simulink subsystem "Read_PX4_Sensors"  (R2025a)
settings: Solver=VariableStepAuto  StartTime=0.0  StopTime=10.0  RelTol=1e-3
libraries: px4uORBlib x8
settings Model: Creator=gurt1  LastModifiedBy=gurt1
settings RTWCC: GPUComputeCapability=3.5

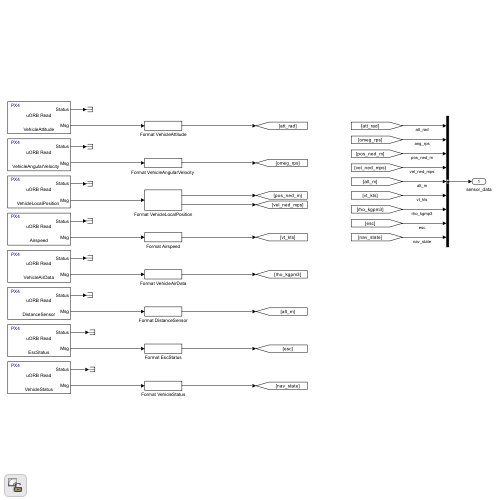
[thumbnail: Simulink's stored preview of the top-level diagram]
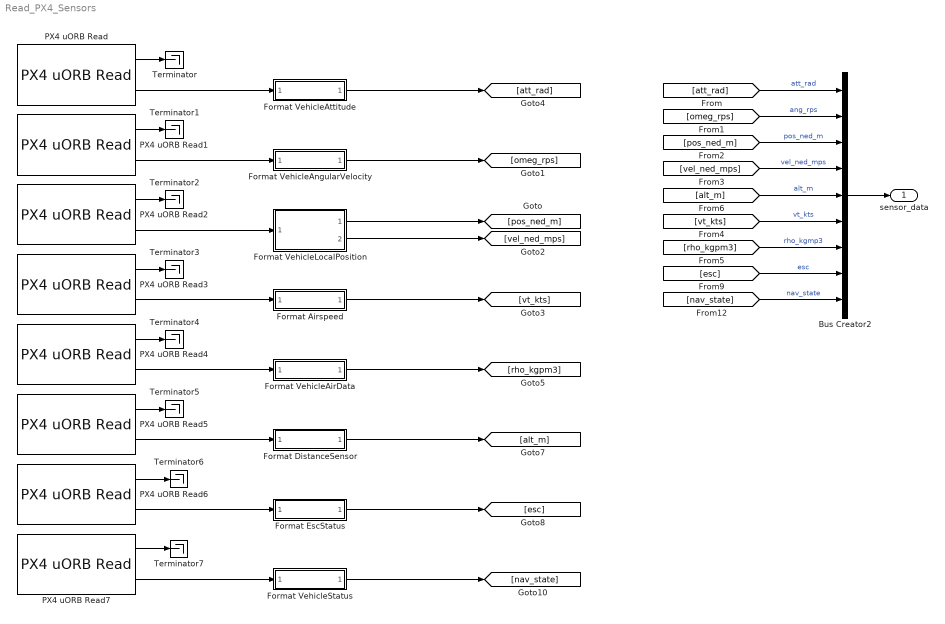
== system Read_PX4_Sensors ==
  Bus Creator2 : BusCreator  Inputs=9
  Format Airspeed : Subsystem
  Format DistanceSensor : Subsystem
  Format EscStatus : Subsystem
  Format VehicleAirData : Subsystem
  "Format VehicleAngularVelocity " : Subsystem
  Format VehicleAttitude : Subsystem
  Format VehicleLocalPosition : Subsystem
  Format VehicleStatus : Subsystem
  PX4 uORB Read : px4uORBlib/PX4 uORB Read  uORBTopic=VehicleAttitude  selectInstance=vehicle_attitude  SampleTime=-1  BlockingMode=off  BlockTimeout=1e-3
  PX4 uORB Read1 : px4uORBlib/PX4 uORB Read  uORBTopic=VehicleAngularVelocity  selectInstance=vehicle_angular_velocity  SampleTime=-1  BlockingMode=off  BlockTimeout=1e-3
  PX4 uORB Read2 : px4uORBlib/PX4 uORB Read  uORBTopic=VehicleLocalPosition  selectInstance=vehicle_local_position  SampleTime=-1  BlockingMode=off  BlockTimeout=1e-3
  PX4 uORB Read3 : px4uORBlib/PX4 uORB Read  uORBTopic=Airspeed  selectInstance=Airspeed  SampleTime=-1  BlockingMode=off  BlockTimeout=1e-3
  PX4 uORB Read4 : px4uORBlib/PX4 uORB Read  uORBTopic=VehicleAirData  selectInstance=VehicleAirData  SampleTime=-1  BlockingMode=off  BlockTimeout=1e-3
  PX4 uORB Read5 : px4uORBlib/PX4 uORB Read  uORBTopic=DistanceSensor  selectInstance=DistanceSensor  SampleTime=-1  BlockingMode=off  BlockTimeout=1e-3
  PX4 uORB Read6 : px4uORBlib/PX4 uORB Read  uORBTopic=EscStatus  selectInstance=EscStatus  SampleTime=-1  BlockingMode=off  BlockTimeout=1e-3
  PX4 uORB Read7 : px4uORBlib/PX4 uORB Read  uORBTopic=VehicleStatus  selectInstance=VehicleStatus  SampleTime=-1  BlockingMode=off  BlockTimeout=1e-3
  Terminator{,1..7} (8 alike) : Terminator
  sensor_data : Outport
  wires:
  PX4 uORB Read/1 -> Terminator/1
  Bus Creator2/1 -> sensor_data/1
  PX4 uORB Read1/1 -> Terminator1/1
  PX4 uORB Read2/1 -> Terminator2/1
  PX4 uORB Read3/1 -> Terminator3/1
  PX4 uORB Read4/1 -> Terminator4/1
  [att_rad] -> Bus Creator2/1  "att_rad"
  [omeg_rps] -> Bus Creator2/2  "ang_rps"
  [pos_ned_m] -> Bus Creator2/3  "pos_ned_m"
  [vel_ned_mps] -> Bus Creator2/4  "vel_ned_mps"
  [vt_kts] -> Bus Creator2/6  "vt_kts"
  [rho_kgpm3] -> Bus Creator2/7  "rho_kgmp3"
  PX4 uORB Read5/1 -> Terminator5/1
  [alt_m] -> Bus Creator2/5  "alt_m"
  PX4 uORB Read6/1 -> Terminator6/1
  [esc] -> Bus Creator2/8  "esc"
  PX4 uORB Read6/2 -> Format EscStatus/1(" ")
  Format EscStatus/1("   ") -> [esc]
  PX4 uORB Read7/1 -> Terminator7/1
  [nav_state] -> Bus Creator2/9  "nav_state"
  PX4 uORB Read/2 -> Format VehicleAttitude/1(" ")
  Format VehicleAttitude/1("  ") -> [att_rad]
  PX4 uORB Read1/2 -> "Format VehicleAngularVelocity "/1(" ")
  "Format VehicleAngularVelocity "/1("  ") -> [omeg_rps]
  PX4 uORB Read2/2 -> Format VehicleLocalPosition/1(" ")
  Format VehicleLocalPosition/1("  ") -> [pos_ned_m]
  Format VehicleLocalPosition/2("   ") -> [vel_ned_mps]
  PX4 uORB Read3/2 -> Format Airspeed/1(" ")
  Format Airspeed/1("  ") -> [vt_kts]
  PX4 uORB Read4/2 -> Format VehicleAirData/1(" ")
  Format VehicleAirData/1("  ") -> [rho_kgpm3]
  PX4 uORB Read5/2 -> Format DistanceSensor/1(" ")
  Format DistanceSensor/1("  ") -> [alt_m]
  PX4 uORB Read7/2 -> Format VehicleStatus/1(" ")
  Format VehicleStatus/1("  ") -> [nav_state]

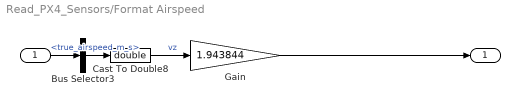
== system Read_PX4_Sensors/Format Airspeed ==
  " " : Inport
  Bus Selector3 : BusSelector  OutputSignals=true_airspeed_m_s
  Cast To Double8 : DataTypeConversion  OutDataTypeStr=double  SaturateOnIntegerOverflow=off  RndMeth=Floor
  Gain : Gain  Gain=1.943844
  "  " : Outport
  wires:
  Cast To Double8/1 -> Gain/1  "vz"
  " "/1 -> Bus Selector3/1
  Gain/1 -> "  "/1
  Bus Selector3/1 -> Cast To Double8/1  "<true_airspeed_m_s>"

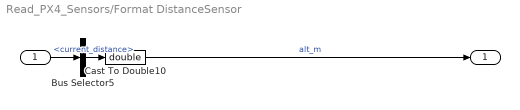
== system Read_PX4_Sensors/Format DistanceSensor ==
  " " : Inport
  Bus Selector5 : BusSelector  OutputSignals=current_distance
  Cast To Double10 : DataTypeConversion  OutDataTypeStr=double  SaturateOnIntegerOverflow=off  RndMeth=Floor
  "  " : Outport
  wires:
  Cast To Double10/1 -> "  "/1  "alt_m"
  Bus Selector5/1 -> Cast To Double10/1  "<current_distance>"
  " "/1 -> Bus Selector5/1

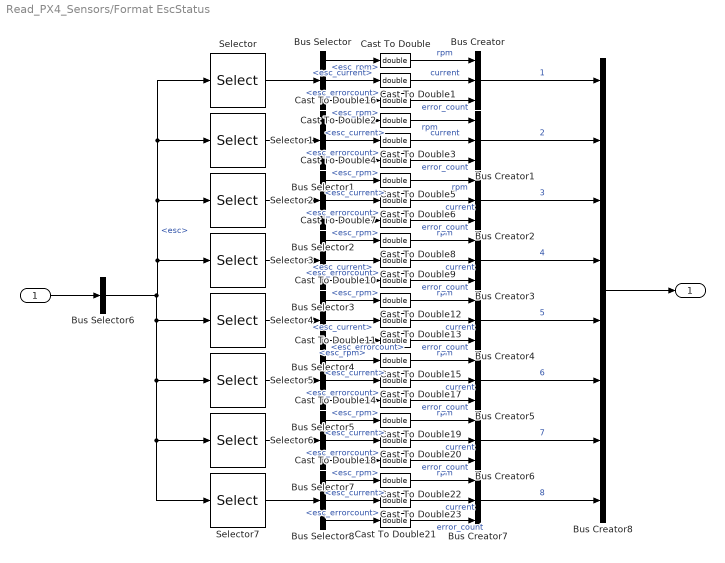
== system Read_PX4_Sensors/Format EscStatus ==
  " " : Inport
  Bus Creator{,1..7} (8 alike) : BusCreator  Inputs=3
  Bus Creator8 : BusCreator  Inputs=8
  Bus Selector{,1..5,7..8} (8 alike) : BusSelector  OutputSignals=esc_rpm,esc_current,esc_errorcount
  Bus Selector6 : BusSelector  OutputSignals=esc
  Cast To Double{,1..23} (24 alike) : DataTypeConversion  OutDataTypeStr=double  SaturateOnIntegerOverflow=off  RndMeth=Floor
  Selector : Selector  InputPortWidth=8  IndexOptions=Index vector (dialog)  Indices=[1]  OutputSizes=1
  Selector1 : Selector  InputPortWidth=8  IndexOptions=Index vector (dialog)  Indices=[2]  OutputSizes=1
  Selector2 : Selector  InputPortWidth=8  IndexOptions=Index vector (dialog)  Indices=[3]  OutputSizes=1
  Selector3 : Selector  InputPortWidth=8  IndexOptions=Index vector (dialog)  Indices=[4]  OutputSizes=1
  Selector4 : Selector  InputPortWidth=8  IndexOptions=Index vector (dialog)  Indices=[5]  OutputSizes=1
  Selector5 : Selector  InputPortWidth=8  IndexOptions=Index vector (dialog)  Indices=[6]  OutputSizes=1
  Selector6 : Selector  InputPortWidth=8  IndexOptions=Index vector (dialog)  Indices=[7]  OutputSizes=1
  Selector7 : Selector  InputPortWidth=8  IndexOptions=Index vector (dialog)  Indices=[8]  OutputSizes=1
  "   " : Outport
  wires:
  Selector3/1 -> Bus Selector3/1
  Bus Creator3/1 -> Bus Creator8/4  "4"
  Cast To Double22/1 -> Bus Creator7/1  "rpm"
  Bus Selector6/1 -> Selector/1, Selector1/1, Selector2/1, Selector3/1, Selector4/1, Selector5/1, Selector6/1, Selector7/1  "<esc>"
  Bus Selector1/1 -> Cast To Double2/1  "<esc_rpm>"
  Cast To Double13/1 -> Bus Creator4/2  "current"
  Bus Selector7/3 -> Cast To Double18/1  "<esc_errorcount>"
  Bus Creator7/1 -> Bus Creator8/8  "8"
  Cast To Double3/1 -> Bus Creator1/2  "current"
  Cast To Double18/1 -> Bus Creator6/3  "error_count"
  Bus Creator2/1 -> Bus Creator8/3  "3"
  Cast To Double15/1 -> Bus Creator5/1  "rpm"
  Cast To Double8/1 -> Bus Creator3/1  "rpm"
  Bus Selector5/3 -> Cast To Double14/1  "<esc_errorcount>"
  Cast To Double16/1 -> Bus Creator/3  "error_count"
  Cast To Double19/1 -> Bus Creator6/1  "rpm"
  Cast To Double9/1 -> Bus Creator3/2  "current"
  " "/1 -> Bus Selector6/1
  Selector2/1 -> Bus Selector2/1
  Cast To Double7/1 -> Bus Creator2/3  "error_count"
  Bus Selector8/1 -> Cast To Double22/1  "<esc_rpm>"
  Selector7/1 -> Bus Selector8/1
  Selector1/1 -> Bus Selector1/1
  Bus Selector2/3 -> Cast To Double7/1  "<esc_errorcount>"
  Bus Selector3/2 -> Cast To Double9/1  "<esc_current>"
  Bus Selector7/2 -> Cast To Double20/1  "<esc_current>"
  Selector6/1 -> Bus Selector7/1
  Cast To Double6/1 -> Bus Creator2/2  "current"
  Selector4/1 -> Bus Selector4/1
  Selector/1 -> Bus Selector/1
  Bus Selector/3 -> Cast To Double16/1  "<esc_errorcount>"
  Bus Creator5/1 -> Bus Creator8/6  "6"
  Bus Selector4/2 -> Cast To Double13/1  "<esc_current>"
  Bus Selector2/2 -> Cast To Double6/1  "<esc_current>"
  Bus Creator6/1 -> Bus Creator8/7  "7"
  Bus Selector8/3 -> Cast To Double21/1  "<esc_errorcount>"
  Bus Creator1/1 -> Bus Creator8/2  "2"
  Selector5/1 -> Bus Selector5/1
  Cast To Double/1 -> Bus Creator/1  "rpm"
  Bus Selector3/1 -> Cast To Double8/1  "<esc_rpm>"
  Bus Selector/1 -> Cast To Double/1  "<esc_rpm>"
  Cast To Double20/1 -> Bus Creator6/2  "current"
  Cast To Double21/1 -> Bus Creator7/3  "error_count"
  Cast To Double12/1 -> Bus Creator4/1  "rpm"
  Bus Selector2/1 -> Cast To Double5/1  "<esc_rpm>"
  Cast To Double4/1 -> Bus Creator1/3  "error_count"
  Bus Selector8/2 -> Cast To Double23/1  "<esc_current>"
  Cast To Double14/1 -> Bus Creator5/3  "error_count"
  Cast To Double2/1 -> Bus Creator1/1  "rpm"
  Cast To Double5/1 -> Bus Creator2/1  "rpm"
  Cast To Double11/1 -> Bus Creator4/3  "error_count"
  Bus Selector4/1 -> Cast To Double12/1  "<esc_rpm>"
  Cast To Double1/1 -> Bus Creator/2  "current"
  Cast To Double17/1 -> Bus Creator5/2  "current"
  Bus Selector1/3 -> Cast To Double4/1  "<esc_errorcount>"
  Bus Creator4/1 -> Bus Creator8/5  "5"
  Bus Selector4/3 -> Cast To Double11/1  "<esc_errorcount>"
  Bus Selector5/2 -> Cast To Double17/1  "<esc_current>"
  Bus Selector3/3 -> Cast To Double10/1  "<esc_errorcount>"
  Bus Selector1/2 -> Cast To Double3/1  "<esc_current>"
  Bus Selector/2 -> Cast To Double1/1  "<esc_current>"
  Cast To Double23/1 -> Bus Creator7/2  "current"
  Bus Creator8/1 -> "   "/1
  Bus Selector5/1 -> Cast To Double15/1  "<esc_rpm>"
  Bus Creator/1 -> Bus Creator8/1  "1"
  Bus Selector7/1 -> Cast To Double19/1  "<esc_rpm>"
  Cast To Double10/1 -> Bus Creator3/3  "error_count"

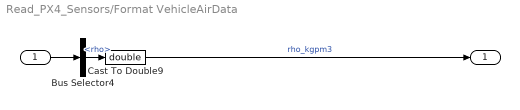
== system Read_PX4_Sensors/Format VehicleAirData ==
  " " : Inport
  Bus Selector4 : BusSelector  OutputSignals=rho
  Cast To Double9 : DataTypeConversion  OutDataTypeStr=double  SaturateOnIntegerOverflow=off  RndMeth=Floor
  "  " : Outport
  wires:
  " "/1 -> Bus Selector4/1
  Cast To Double9/1 -> "  "/1  "rho_kgpm3"
  Bus Selector4/1 -> Cast To Double9/1  "<rho>"

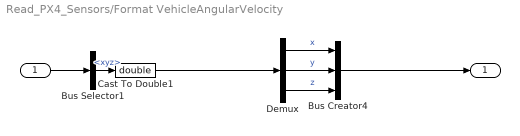
== system Read_PX4_Sensors/Format VehicleAngularVelocity  ==
  " " : Inport
  Bus Creator4 : BusCreator  Inputs=3
  Bus Selector1 : BusSelector  OutputSignals=xyz
  Cast To Double1 : DataTypeConversion  OutDataTypeStr=double  SaturateOnIntegerOverflow=off  RndMeth=Floor
  Demux : Demux  Outputs=3
  "  " : Outport
  wires:
  Bus Creator4/1 -> "  "/1
  Demux/3 -> Bus Creator4/3  "z"
  Bus Selector1/1 -> Cast To Double1/1  "<xyz>"
  Demux/1 -> Bus Creator4/1  "x"
  Demux/2 -> Bus Creator4/2  "y"
  Cast To Double1/1 -> Demux/1
  " "/1 -> Bus Selector1/1

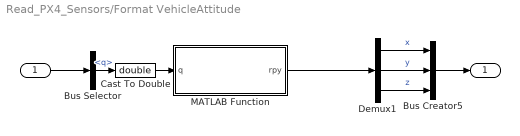
== system Read_PX4_Sensors/Format VehicleAttitude ==
  " " : Inport
  Bus Creator5 : BusCreator  Inputs=3
  Bus Selector : BusSelector  OutputSignals=q
  Cast To Double : DataTypeConversion  OutDataTypeStr=double  SaturateOnIntegerOverflow=off  RndMeth=Floor
  Demux1 : Demux  Outputs=3
  MATLAB Function : MATLAB Function  TreatAsAtomicUnit=on
  "  " : Outport
  wires:
  Bus Creator5/1 -> "  "/1
  Bus Selector/1 -> Cast To Double/1  "<q>"
  Demux1/1 -> Bus Creator5/1  "x"
  Cast To Double/1 -> MATLAB Function/1(q)
  Demux1/2 -> Bus Creator5/2  "y"
  MATLAB Function/1(rpy) -> Demux1/1
  Demux1/3 -> Bus Creator5/3  "z"
  " "/1 -> Bus Selector/1

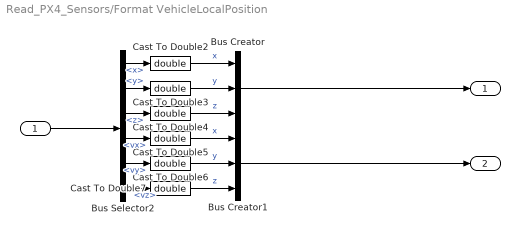
== system Read_PX4_Sensors/Format VehicleLocalPosition ==
  " " : Inport
  Bus Creator : BusCreator  Inputs=3
  Bus Creator1 : BusCreator  Inputs=3
  Bus Selector2 : BusSelector  OutputSignals=x,y,z,vx,vy,vz
  Cast To Double{2..7} (6 alike) : DataTypeConversion  OutDataTypeStr=double  SaturateOnIntegerOverflow=off  RndMeth=Floor
  "  " : Outport
  "   " : Outport  Port=2
  wires:
  " "/1 -> Bus Selector2/1
  Bus Creator/1 -> "  "/1
  Cast To Double5/1 -> Bus Creator1/1  "x"
  Cast To Double6/1 -> Bus Creator1/2  "y"
  Bus Selector2/4 -> Cast To Double5/1  "<vx>"
  Cast To Double2/1 -> Bus Creator/1  "x"
  Bus Selector2/3 -> Cast To Double4/1  "<z>"
  Bus Creator1/1 -> "   "/1
  Cast To Double7/1 -> Bus Creator1/3  "z"
  Bus Selector2/5 -> Cast To Double6/1  "<vy>"
  Cast To Double3/1 -> Bus Creator/2  "y"
  Bus Selector2/1 -> Cast To Double2/1  "<x>"
  Bus Selector2/6 -> Cast To Double7/1  "<vz>"
  Cast To Double4/1 -> Bus Creator/3  "z"
  Bus Selector2/2 -> Cast To Double3/1  "<y>"

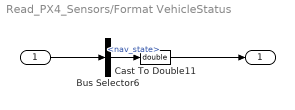
== system Read_PX4_Sensors/Format VehicleStatus ==
  " " : Inport
  Bus Selector6 : BusSelector  OutputSignals=nav_state
  Cast To Double11 : DataTypeConversion  OutDataTypeStr=double  SaturateOnIntegerOverflow=off  RndMeth=Floor
  "  " : Outport
  wires:
  " "/1 -> Bus Selector6/1
  Cast To Double11/1 -> "  "/1
  Bus Selector6/1 -> Cast To Double11/1  "<nav_state>"

== matlab function Read_PX4_Sensors/Format VehicleAttitude/MATLAB Function ==
  data: q input; rpy output
function rpy = q2euler_angles(q)

rpy = q2euler_angles(q);
